simulink model "voltify_simscape_model"  (R2024b)
settings: Solver=VariableStepAuto  StartTime=0.0  StopTime=1  RelTol=1e-3
libraries: fl_lib x6, nesl_utility x5
settings Model: Creator=BillBeverley  LastModifiedBy=BillBeverley

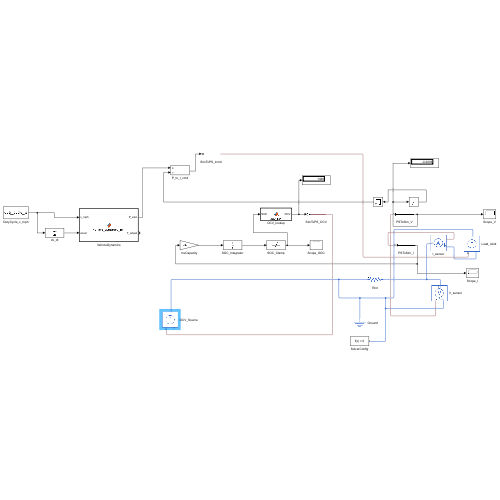
[thumbnail: Simulink's stored preview of the top-level diagram]
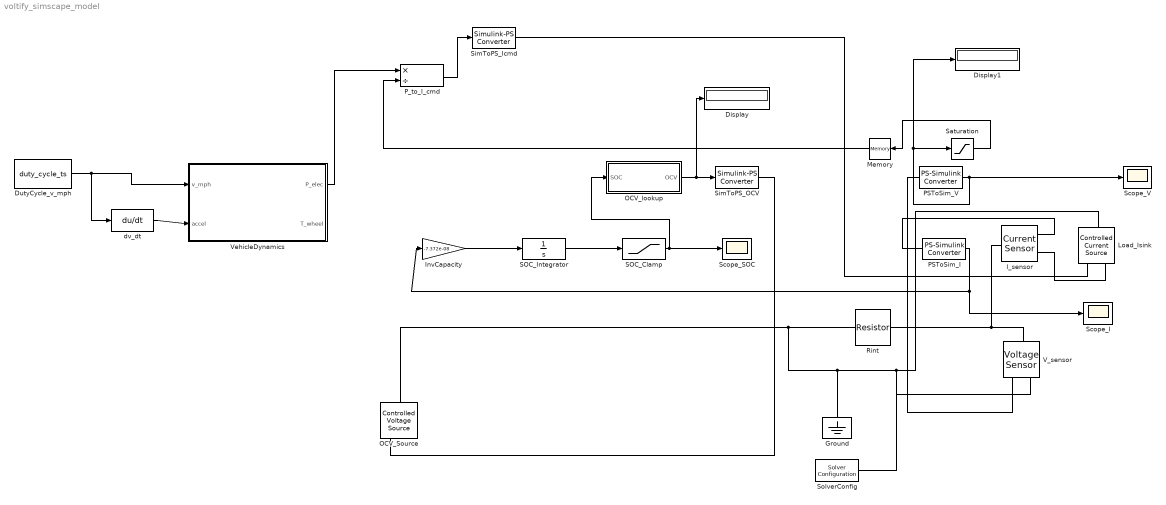
== system voltify_simscape_model ==
  Display : Display
  Display1 : Display
  DutyCycle_v_mph : FromWorkspace  VariableName=duty_cycle_ts
  Ground : fl_lib/Electrical/Electrical Elements/Electrical Reference
  I_sensor : fl_lib/Electrical/Electrical Sensors/Current Sensor
  InvCapacity : Gain  Gain=-7.372e-08
  Load_Isink : fl_lib/Electrical/Electrical Sources/Controlled Current Source
  Memory : Memory  InitialCondition=1447.68
  OCV_Source : fl_lib/Electrical/Electrical Sources/Controlled Voltage Source
  OCV_lookup : MATLAB Function  TreatAsAtomicUnit=on
  PSToSim_I : nesl_utility/PS-Simulink Converter  PhysicalDomain=network_engine_domain  SubClassName=ps_output  LeftPortType=input  RightPortType=output  PseudoPeriodic=off  Frequencies=[]  VectorFormat=inherit  Unit=inherit  AffineConversion=off
  PSToSim_V : nesl_utility/PS-Simulink Converter  PhysicalDomain=network_engine_domain  SubClassName=ps_output  LeftPortType=input  RightPortType=output  PseudoPeriodic=off  Frequencies=[]  VectorFormat=inherit  Unit=inherit  AffineConversion=off
  P_to_I_cmd : Product  Inputs=*/
  Rint : fl_lib/Electrical/Electrical Elements/Resistor  R=0.05 Ohm  i_specify=off  i_priority=None  i=0 A  i_nominal_specify=off  i_nominal_value=1  i_nominal_unit=A  v_specify=off  v_priority=None  v=0 V  v_nominal_specify=off  v_nominal_value=1  v_nominal_unit=V
  SOC_Clamp : Saturate  UpperLimit=1  LowerLimit=0
  SOC_Integrator : Integrator  InitialCondition=0.9
  Saturation : Saturate  UpperLimit=1500  LowerLimit=1000
  Scope_I : Scope
  Scope_SOC : Scope
  Scope_V : Scope
  SimToPS_Icmd : nesl_utility/Simulink-PS Converter  PhysicalDomain=network_engine_domain  SubClassName=ps_input  LeftPortType=input  RightPortType=output  PseudoPeriodic=off  Frequencies=[]  NoiseDistribution=none  NoiseParameters=[]  Unit=1  AffineConversion=off  FilteringAndDerivatives=provide  SimscapeFilterOrder=1  InputFilterTimeConstant=0.001  UdotUserProvided=0
  SimToPS_OCV : nesl_utility/Simulink-PS Converter  PhysicalDomain=network_engine_domain  SubClassName=ps_input  LeftPortType=input  RightPortType=output  PseudoPeriodic=off  Frequencies=[]  NoiseDistribution=none  NoiseParameters=[]  Unit=1  AffineConversion=off  FilteringAndDerivatives=provide  SimscapeFilterOrder=1  InputFilterTimeConstant=0.001  UdotUserProvided=0
  SolverConfig : nesl_utility/Solver Configuration  PhysicalDomain=network_engine_domain  SubClassName=solver  LeftPortType=input  RightPortType=generic  Tones=[]  Harmonics=[]  SimulateNoise=off  Profile=off  UseLocalSampling=off  EnableSwitchedLinearOptims=on  FrequencyDomain=off  UseCCode=off  RelTol=0.001  AbsTol=0.001  MinStep=1e-09  ToWorkspace=off  RevertToSquareIcSolve=off  NumHomotopyIterations=100  PhasorMode=off  PhasorModeNumHarmonics=1  ConsistencySolver=NEWTON_XTOL_AFTER_FTOL  IndexReductionMethod=DerivativeReplacement  DoDC=off  ResidualTolerance=1e-09  ConsistencyTolSource=GLOBAL  ConsistencyAbsTol=0.001  ConsistencyRelTol=0.001  ConsistencyTolFactor=0.001  UseLocalSolver=off  LocalSolverChoice=NE_BACKWARD_EULER_ADVANCER  ResolveIndetEquations=on  FunctionEvalNumThread=1  LocalSolverSampleTime=0.001  DoFixedCost=off  MaxNonlinIter=3  MaxModeIter=2  ComputeImpulses=off  ImpulseIterations=2  LinearAlgebra=auto  LinearAlgebraNumThread=0  EquationFormulation=NE_TIME_EF  DelaysMemoryBudget=1024  AutomaticFiltering=on  FilteringTimeConstant=0.001  PartitionStorageMethod=AS_NEEDED  PartitionMemoryBudget=1024  PartitionMethod=ROBUST  MultibodyUseLocalSolver=off  MultibodyLocalSolverChoice=ODE1  MultibodyLocalSolverSampleTime=0.001
  V_sensor : fl_lib/Electrical/Electrical Sensors/Voltage Sensor
  VehicleDynamics : MATLAB Function  TreatAsAtomicUnit=on
  dv_dt : Derivative
  wires:
  DutyCycle_v_mph/1 -> VehicleDynamics/1(v_mph), dv_dt/1
  dv_dt/1 -> VehicleDynamics/2(accel)
  VehicleDynamics/1(P_elec) -> P_to_I_cmd/1
  PSToSim_V/1 -> Display1/1, Saturation/1, Scope_V/1
  P_to_I_cmd/1 -> SimToPS_Icmd/1
  PSToSim_I/1 -> InvCapacity/1, Scope_I/1
  InvCapacity/1 -> SOC_Integrator/1
  SOC_Integrator/1 -> SOC_Clamp/1
  SOC_Clamp/1 -> OCV_lookup/1(SOC), Scope_SOC/1
  OCV_lookup/1(OCV) -> Display/1, SimToPS_OCV/1
  Memory/1 -> P_to_I_cmd/2
  Saturation/1 -> Memory/1
  connections:
  OCV_Source/LConn1 -- Rint/LConn1 -- SolverConfig/RConn1 -- V_sensor/RConn2 -- Load_Isink/LConn1 -- Ground/LConn1
  Rint/RConn1 -- V_sensor/LConn1 -- I_sensor/LConn1
  SimToPS_OCV/RConn1 -- OCV_Source/RConn1
  V_sensor/RConn1 -- PSToSim_V/LConn1
  I_sensor/RConn2 -- Load_Isink/RConn2
  SimToPS_Icmd/RConn1 -- Load_Isink/RConn1
  I_sensor/RConn1 -- PSToSim_I/LConn1

== matlab function voltify_simscape_model/VehicleDynamics ==
  data: v_mph input; P_elec output; accel input; T_wheel output
function [P_elec, T_wheel] = vehicle_dynamics_fcn(v_mph, accel)
%#codegen
mass = 122469.8400; g = 9.81; Crr = 0.00200; Cd = 0.800; A = 10.000; rho = 1.225;
r_wheel = 0.50800; gear_ratio = 4.1300; eta_m = 0.9200; eta_r = 0.8500;
v = v_mph * 0.44704;
F_roll = sign(v) * mass * g * Crr;
F_aero = 0.5 * rho * Cd * A * v * abs(v);
F_acc  = mass * accel;
F_trac = F_acc + F_roll + F_aero;
T_wheel = F_trac * r_wheel;
P_mech = F_trac * v;
if P_mech >= 0
    P_elec = P_mech / eta_m;
else
    P_elec = P_mech * eta_r;
end
end

== matlab function voltify_simscape_model/OCV_lookup ==
  data: SOC input; OCV output
function OCV = ocv_fcn(SOC)
%#codegen
Vmin = 1185.60; Vmax = 1476.80;
OCV = Vmin + (Vmax-Vmin)*SOC; % linear placeholder -- replace with LFP lookup table
end
